simulink model "Underwaterproject1"  (R2018b)
settings: Solver=VariableStepAuto  StartTime=0.0  StopTime=3.6  RelTol=1e-3
libraries: SignalEditorBlockLib x1, simulink_extras x1
settings Model: Creator=ali  LastModifiedBy=Ali

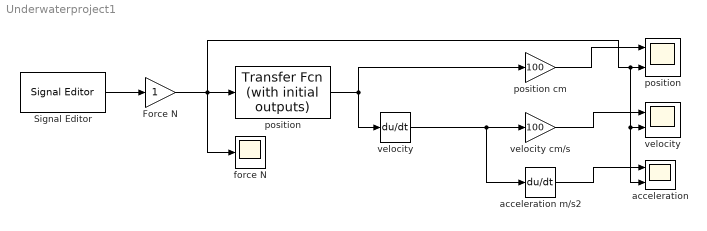
== system Underwaterproject1 ==
  Force N : Gain
  Signal Editor : SignalEditorBlockLib/Signal Editor  FileName=C:\Users\ali\Desktop\Underwaterproject1\zigzag.mat  ActiveScenario=ZIGZAG  ActiveSignal=Signal zigzag  IsBus=off  OutputBusObjectStr=Bus: BusObject  SampleTime=0.1  ZeroCross=off  OutputAfterFinalValue=Setting to zero  Unit=inherit
  "acceleration " : Scope  NumInputPorts=2
  acceleration m/s2 : Derivative
  "force N " : Scope
  position : simulink_extras/Additional Linear/Transfer Fcn (with initial outputs)  N=[1]  D=[1 10 100]  Y0=0  U0=0
  "position " : Scope  NumInputPorts=2
  position cm : Gain  Gain=100
  velocity : Derivative
  "velocity " : Scope  NumInputPorts=2
  velocity cm/s : Gain  Gain=100
  wires:
  acceleration m/s2/1 -> "acceleration "/1
  velocity/1 -> velocity cm/s/1, acceleration m/s2/1
  Signal Editor/1 -> Force N/1
  Force N/1 -> "position "/2, "acceleration "/2, "velocity "/2, "force N "/1, position/1
  position cm/1 -> "position "/1
  velocity cm/s/1 -> "velocity "/1
  position/1 -> velocity/1, position cm/1
